simulink model "compr"  (R2018a)
settings: Solver=VariableStepAuto  StartTime=0.0  StopTime=100  RelTol=1e-3
libraries: dspvision x2, dspsnks4 x1, audiodynamicrange x1
settings Model: Creator=116983  LastModifiedBy=stefa

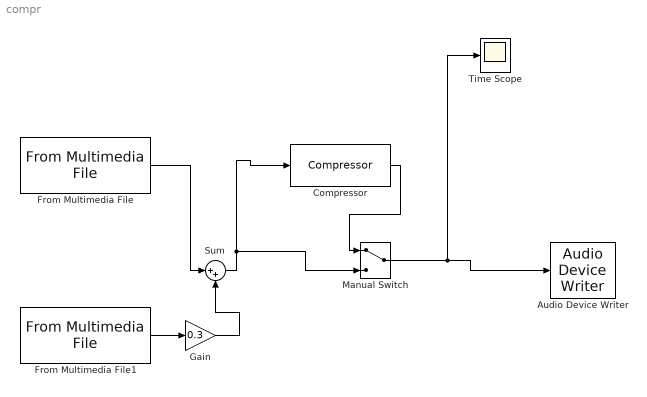
== system compr ==
  Audio Device Writer : dspsnks4/Audio Device Writer  Driver=DirectSound  Device=Default  InheritSampleRate=on  SampleRate=44100  BitDepth=16-bit integer  BufferSize=4096  NumBuffers=10  DefaultOutputChannelMapping=on  OutputChannelMapping=1:2  OutputNumUnderrunSamples=off  DriverIdx=1  DeviceWarnFlag=''
  Compressor : audiodynamicrange/Compressor  ThresholdPort=off  Threshold=-27.500  RatioPort=off  Ratio=50.0  KneeWidthPort=off  KneeWidth=3.600  AttackTimePort=off  AttackTime=0.0  ReleaseTimePort=off  ReleaseTime=0.120  MakeUpGainMode=Property  MakeUpGain=19.920  InheritSampleRate=on  SampleRate=44100  outputGain=off  SimulateUsing=Interpreted execution
      settings: SourceProductName=Audio System Toolbox  SourceProductBaseCode=AU
  From Multimedia File : dspvision/From Multimedia File  inputFilename=C:\Users\stefa\Dropbox\magistrale\Bernardini\algoritmi_shot_gianca\g3sg1-1.wav  loop=on  numPlays=inf  outputStreams=Audio only  videoDataType=single  audioDataType=double  inheritSampleTime=on  userDefinedSampleTime=1/30  noAudioOutput=off  isIntensityVideo=off  fourcc=RGB  colorVideoFormat=Separate color signals  outputEOF=off  dataOrg=Column-major  audioFrameSize=1024  computeAudioFrameSize=off  outSamplingMode=Sample based
      settings: SourceProductBaseCode=VP
  From Multimedia File1 : dspvision/From Multimedia File  inputFilename=C:\Users\stefa\Dropbox\magistrale\Bernardini\audio\divina_commedia.wav  loop=on  numPlays=inf  outputStreams=Audio only  videoDataType=single  audioDataType=double  inheritSampleTime=on  userDefinedSampleTime=1/30  noAudioOutput=off  isIntensityVideo=off  fourcc=RGB  colorVideoFormat=Separate color signals  outputEOF=off  dataOrg=Column-major  audioFrameSize=1024  computeAudioFrameSize=off  outSamplingMode=Sample based
      settings: SourceProductBaseCode=VP
  Gain : Gain  Gain=0.3
  Manual Switch : ManualSwitch
  Sum : Sum  Inputs=|++
  Time Scope : Scope
  wires:
  Sum/1 -> Manual Switch/2, Compressor/1
  From Multimedia File/1 -> Sum/1
  From Multimedia File1/1 -> Gain/1
  Compressor/1 -> Manual Switch/1
  Manual Switch/1 -> Time Scope/1, Audio Device Writer/1
  Gain/1 -> Sum/2
